simulink model "sim_002"  (R2015b)
settings: Solver=ode45  StartTime=0.0  StopTime=180  MaxStep=0.26  RelTol=1e-3
settings Model: Creator=nandomgu  LastModifiedBy=nandomgu
settings DataIOCC: OutputOption=SpecifiedOutputTimes  ReturnWorkspaceOutputsName=simoutput

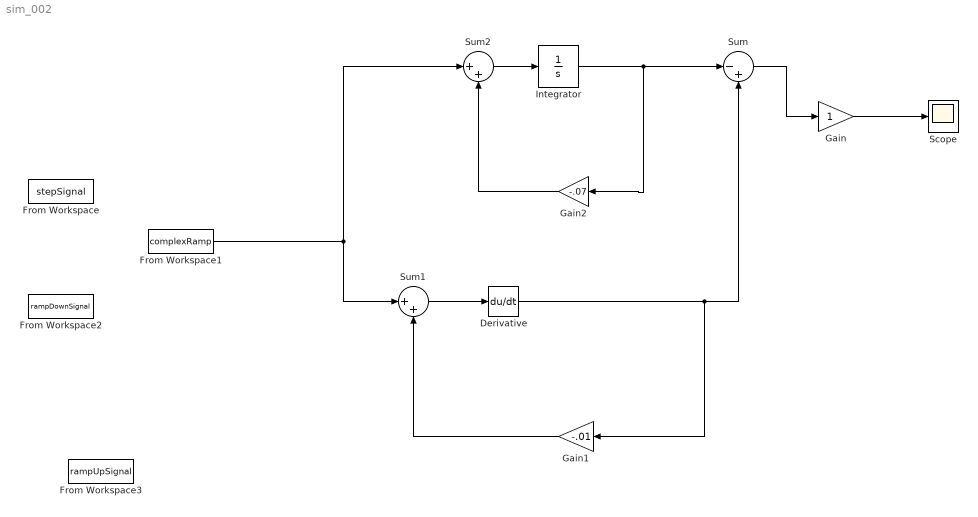
== system sim_002 ==
  Derivative : Derivative
  From Workspace : FromWorkspace  VariableName=stepSignal  OutDataTypeStr=double
  From Workspace1 : FromWorkspace  VariableName=complexRamp  OutDataTypeStr=double
  From Workspace2 : FromWorkspace  VariableName=rampDownSignal  OutDataTypeStr=double
  From Workspace3 : FromWorkspace  VariableName=rampUpSignal  OutDataTypeStr=double
  Gain : Gain
  Gain1 : Gain  Gain=-.01
  Gain2 : Gain  Gain=-.07
  Integrator : Integrator
  Scope : Scope
  Sum : Sum  Inputs=|-+
  Sum1 : Sum  Inputs=|++
  Sum2 : Sum  Inputs=|++
  wires:
  Integrator/1 -> Gain2/1, Sum/1
  Gain/1 -> Scope/1
  Sum/1 -> Gain/1
  From Workspace1/1 -> Sum1/1, Sum2/1
  Sum2/1 -> Integrator/1
  Gain2/1 -> Sum2/2
  Derivative/1 -> Sum/2, Gain1/1
  Gain1/1 -> Sum1/2
  Sum1/1 -> Derivative/1
